simulink model "Wanchao_shuttlecock"  (Simulink 7.8)
settings: Solver=ode4  StartTime=0.0  StopTime=inf  FixedStep=sample_time  RelTol=1e-3
InitFcn:
  | sample_time=0.005;%0.004;%0.0025;%0.02;
  | DeltaT = 0.02;
  | g = 9.81;
  | H0 = g%0.3165;
  | Kl = 1;
  | 
  | Omega_r = 1.6;%for Horizontal reference
  | Zeta_r = 0.7; %for Horizontal reference
  | Omega = 1.8;%for Horizontal Control
  | Zeta = 0.5;    %for Horizontal Control
  | 
  | Omega_h_r = 2.5; %for vertical reference
  | Zeta_h_r = 0.8;  %for vertical reference
  | Omega_h = 2.7;    %for vertical control
  | Zeta_h = 0.8;         %for vertical control
  | PI=pi;
  | 
  | Mass = 1.1;
  | Acc_Max = 4;
  | Acc_Max_h = 4;
  | 
  | Max_RP = 60;
  | 
  | load MaoBi_Oct04_2_int.mat
  | MB_Interp.time = [];
undefined symbols (not defined in the file or in its folder): DiscIntNeverNeededParam
libraries: simulink x7, dspadpt3 x3, X330_Control x2, X400_Control x1
(part 2 of 2)

== stateflow chart Planning/Trajectory Logic/UAV SF ==
  state Landing
    state Descending
      en:PosDesired = Pos;
      du:PosDesired[2] = (PerchPos[2]- PosDesired[2])*1*DeltaT + PosDesired[2] ;
    state CutThrottle
      du:HoverThrottle = (0 - HoverThrottle)*3*DeltaT + HoverThrottle ;
    (default) -> Descending
    Descending -> CutThrottle : [Pos[2] > (PerchPos[2]-0.1)]
  state Airborne
    state TakeOff
      du:HoverThrottle = (H0 - HoverThrottle)*3*DeltaT + HoverThrottle ;
    state Initialization
      du:PosDesired=InitialPos;
    state SafyHover
      en:PosDesired = Pos; PosDesired[2]=-1.2;
    state Prelanding
      en:PosDesired=InitialPos ;
    state Descent
      en:PosDesired[2] = PerchPos[2]-0.15;
    state TrajEst
      state DAQ [parallel]
        en:i=0;
        du:PosShtlck[i,:]=Shuttlecock;i++;
        settings: executionOrder=1
      state Estimation [parallel]
        en:PosEst=TrajEst(PosShtl,H);
        du:PosDesired=PosEst;
        settings: executionOrder=2
      (junction 23) -> DAQ [order 1] : [(Shuttlecock[2]-H<-0.4)|(Shuttlecock[5]<0)]{i=0;}
      DAQ -> (junction 23) : [i==5]{PosShtl=PosShtlck;}
      (junction 23) -> Estimation [order 2]
      (default) -> DAQ
    (default) -> TakeOff : {PosDesired = Pos;PosDesired[2] =-1.2;}
    Initialization -> SafyHover [order 2] : [RC[5] > 0]
    TakeOff -> Initialization : after(3,sec)
    SafyHover -> Prelanding : after(3, sec)
    Prelanding -> Descent : [PerchError < 0.01]
    Initialization -> TrajEst [order 1] : [(abs(Shuttlecock[0])<1)&(Shuttlecock[1]<2.8)&(Shuttlecock[2]<H)]
    TrajEst -> SafyHover : [(RC[5] > 0)]
  (default) -> Landing : {HoverThrottle = 0;}
  Airborne -> Landing : [RC[6] < -0.5]
  Landing -> Airborne : [RC[6] > 0.5]
  data: Shuttlecock function_input double; PosEst function_output double; H function_input double; PosDesired output double size=4; HoverThrottle output double size=1; Mode output uint8 size=1; RC input double size=8; Pos input double size=4; PerchPos input double size=4; DeltaT parameter double size=1; H0 parameter double size=1; Kl parameter double size=1; VelCmd local double size=2 =0; PWM output double; PerchError input double; PI parameter double size=1; Shuttlecock input double; InitialPos constant double size=3 =[0,-1,-1.2]; i local double =0; PosShtlck local double; PosEst output double; PosShtl local double; H constant double =-1.3
  data H settings: description=Target Height
  events: trigger local EITHER_EDGE_EVENT
  function PosEst=TrajEst(Shuttlecock,H):
    | function PosEst=TrajEst(Shuttlecock,H)
    | 
    | n=length(Shuttlecock(:,1));
    | 
    | sgn=sign(mean(Shuttlecock(:,4)));
    | dx=sgn*0.01;
    | x=Shuttlecock(1,1):dx:sgn;
    | y=Shuttlecock(2,1):-0.01:-1.5;
    | 
    | tr_zx=polyval(polyfit(Shuttlecock(:,1),Shuttlecock(:,3),2),x);
    | tr_zy=polyval(polyfit(Shuttlecock(:,2),Shuttlecock(:,3),2),y);
    | 
    | [~,kx]=min(abs(tr_zx-H));
    | [~,ky]=min(abs(tr_zy-H));
    | 
    | xe=x(kx);
    | ye=y(ky);
    | 
    | PosEst=[xe,ye,H-0.1];
